simulink model "Model_Vehicle1D_Custom_24b"  (R2024b)
settings: Solver=VariableStepAuto  StartTime=0.0  StopTime=300  RelTol=1e-3
libraries: fl_lib x6, nesl_utility x4, sdl_lib x2
settings Model: Creator=isaacito  LastModifiedBy=isaacito
settings DataIOCC: DSMLogging=off
settings SimscapeCC: SimscapeLogType=all  SimscapeLogSimulationStatistics=on  SimscapeLogLimitData=off

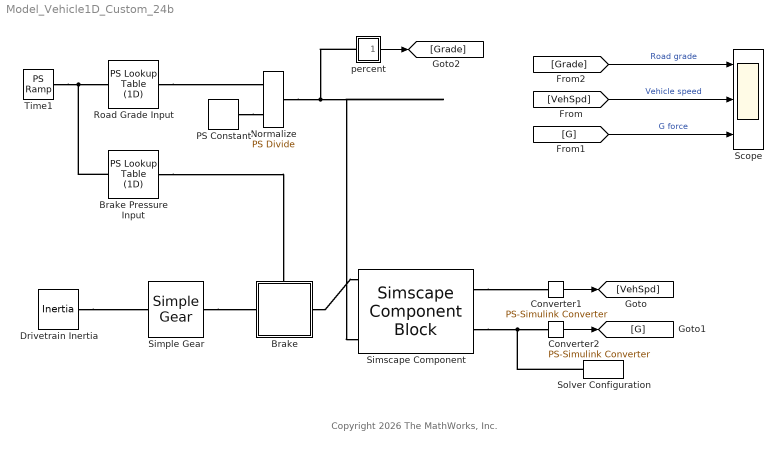
== system Model_Vehicle1D_Custom_24b ==
  note: Copyright 2026 The MathWorks, Inc.
  Brake : Subsystem
      settings: PortSchema="{\"entries\":[{\"content\":{\"sides\":[{\"content\":{\"connectorIds\":[\"LConn1\"]},\"type\":\"ConnectorPlacement.EquallySpacedRectSide\",\"uuid\":\"c6b073dd-2713-4a5b-85ee-4b5913294757\"},{\"content\":{\"connectorIds\":[\"RConn1\"],\"side\":\"RIGHT\"},\"type\":\"ConnectorPlacement.EquallySpacedRectSide\",\"uuid\":\"bfc45b1f-17ac-472b-87f9-2453469bccb5\"},{\"content\":{\"connectorIds\":[\"LConn2\"],\"side\":\"TOP\"},\"type\":\"ConnectorPlacement.EquallySpacedRectSide\",\"uuid\":\"4f05775c-3f1a-4bd9-8953-8138b3f9abd3\"}]},\"type\":\"ConnectorPlacement.EquallySpacedConnector\",\"uuid\":\"6aab441d-31a0-4c85-b942-993fc4aff852\"}],\"packageUris\":[\"http://schema.mathworks.com/mf0/Connector/R2020b\"],\"version\":\"1.0\"}"
  Brake Pressure Input : fl_lib/Physical Signals/Lookup Tables/PS Lookup Table (1D)  x=[0 1 2] s  f=[0 0 0] Pa  interp_method=simscape.enum.interpolation.smooth  extrap_method=simscape.enum.extrapolation.nearest
  Converter1 : nesl_utility/PS-Simulink Converter  PhysicalDomain=network_engine_domain  SubClassName=ps_output  LeftPortType=input  RightPortType=output  PseudoPeriodic=off  Frequencies=[]  VectorFormat=inherit  Unit=km/hr  AffineConversion=off
  Converter2 : nesl_utility/PS-Simulink Converter  PhysicalDomain=network_engine_domain  SubClassName=ps_output  LeftPortType=input  RightPortType=output  PseudoPeriodic=off  Frequencies=[]  VectorFormat=inherit  Unit=1  AffineConversion=off
  Drivetrain Inertia : fl_lib/Mechanical/Rotational Elements/Inertia  inertia=20*0.1^2 kg*m^2  num_ports=foundation.enum.numPorts2.one  w_specify=off  w_priority=High  w=0 rad/s  w_nominal_specify=off  w_nominal_value=1  w_nominal_unit=rad/s  t_specify=off  t_priority=None  t=0 N*m  t_nominal_specify=off  t_nominal_value=1  t_nominal_unit=N*m
  Normalize : fl_lib/Physical Signals/Functions/PS Divide
  PS Constant : fl_lib/Physical Signals/Sources/PS Constant  constant=100
      settings: AttributesFormatString=%<constant>
  Road Grade Input : fl_lib/Physical Signals/Lookup Tables/PS Lookup Table (1D)  Description=|  x=[0, 2.5, 5, 10, 25, 40, 80, 85, 90, 110, 130, 165, 200] s  f=[0, 0, 0, -10, -10, -10, 0, 0, 0, 5, 0, 0, 0]  interp_method=simscape.enum.interpolation.smooth  extrap_method=simscape.enum.extrapolation.nearest
      | % This text was automatically inserted by Signal Util.
      | % SignalDesignMatrixStart
      | [0 5 0; 10 40 -10; 80 90 0;
      |  110 nan 5; 130 200 0]
      | 
      | % SignalDesignMatrixEnd
  Scope : Scope  NumInputPorts=3
  Simple Gear : sdl_lib/Gears/Simple Gear  ratio=1/10  rotation_direction=sdl.enum.shaftOutputDirection.same  friction_model=sdl.enum.gear_efficiencies_load.off  T_noload=0.1 N*m  T_nom=5 N*m  efficiency_nom=0.8  efficiency=0.8  temperature_TLU=[280, 300, 320] K  load_TLU=[1, 5, 10] N*m  efficiency_TLU=[.95, .9, .85]  efficiency_TLU2=[.85, .8, .75; .95, .9, .85; .85, .8, .7]  w_thr=0.01 rad/s  pwr_thr=0.001 W  enable_backlash=false  hardstop_model=simscape.enum.hardstop.smooth  backlash_distance=1e-3 mm  r_base=0.1 m  transition=1e-4 mm  backlash_stiffness=1e6 N/m  backlash_damping=1e3 N*s/m  coeff_rest=0.7  v_tol=0.001 m/s  f_tol=0.001 N  mu_visc=[0, 0] N*m*s/rad  thermal_mass=50 J/K  temperature_specify=off  temperature_priority=High  temperature=300 K  temperature_nominal_specify=off  temperature_nominal_value=1  temperature_nominal_unit=K  x_backlash_specify=off  x_backlash_priority=None  x_backlash=0 mm  x_backlash_nominal_specify=off  x_backlash_nominal_value=1  x_backlash_nominal_unit=mm  f_hardstop_specify=off  f_hardstop_priority=None  f_hardstop=0 N  f_hardstop_nominal_specify=off  f_hardstop_nominal_value=1  f_hardstop_nominal_unit=N  v_backlash_specify=off  v_backlash_priority=None  v_backlash=0 m/s  v_backlash_nominal_specify=off  v_backlash_nominal_value=1  v_backlash_nominal_unit=m/s
      settings: AttributesFormatString=%<ratio>
  Simscape Component : SimscapeComponentBlock  SourceFile=Vehicle1D_Custom  ComponentPath=Vehicle1D_Custom  ComponentVariants="[\"Vehicle1D_Custom\"]"  ComponentVariantNames="[\"Vehicle1D_Custom\"]"  ClassName=Vehicle1D_Custom  SchemaVersion=1  grav=9.81 m/s^2  M_e=1500 kg  R_tire=0.3 m  A_rl=120 N  B_rl=0 N*hr/km  C_rl=0.03 N*hr^2/km^2  V_1=0.1 km/hr  w_1=0.1 rpm  V_x_specify=off  V_x_priority=High  V_x=0 km/hr  V_x_nominal_specify=off  V_x_nominal_value=1  V_x_nominal_unit=km/hr
      settings: CopyFcn=simscape.engine.sli.internal.componentblockcallback(gcbh,'COPY')  PreCopyFcn=simscape.engine.sli.internal.componentblockcallback(gcbh,'PRECOPY')  PreDeleteFcn=simscape.engine.sli.internal.componentblockcallback(gcbh,'PREDELETE')  InternalSimscapePortConfiguration="{\"Bottom\":[],\"Left\":[{\"id\":\"Axle\",\"label\":\"Axle\",\"type\":\"foundation.mechanical.rotational.rotational\"}],\"Right\":[{\"id\":\"v_out\",\"label\":\"V\",\"type\":\"output\"},{\"id\":\"G\",\"label\":\"G\",\"type\":\"output\"}],\"Top\":[{\"id\":\"brkF\",\"label\":\"Brake\",\"type\":\"input\"},{\"id\":\"grade_norm\",\"label\":\"Grade\",\"type\":\"input\"}]}"
      mask Type: Custom Longitudinal Vehicle
  Solver Configuration : nesl_utility/Solver Configuration  PhysicalDomain=network_engine_domain  SubClassName=solver  LeftPortType=input  RightPortType=generic  Tones=[]  Harmonics=[]  SimulateNoise=off  Profile=off  UseLocalSampling=off  EnableSwitchedLinearOptims=on  FrequencyDomain=off  UseCCode=off  RelTol=0.001  AbsTol=0.001  MinStep=1e-09  ToWorkspace=off  RevertToSquareIcSolve=off  NumHomotopyIterations=100  PhasorMode=off  PhasorModeNumHarmonics=1  ConsistencySolver=NEWTON_XTOL_AFTER_FTOL  IndexReductionMethod=DerivativeReplacement  DoDC=off  ResidualTolerance=1e-09  ConsistencyTolSource=GLOBAL  ConsistencyAbsTol=0.001  ConsistencyRelTol=0.001  ConsistencyTolFactor=0.001  UseLocalSolver=off  LocalSolverChoice=NE_BACKWARD_EULER_ADVANCER  ResolveIndetEquations=on  FunctionEvalNumThread=1  LocalSolverSampleTime=0.001  DoFixedCost=off  MaxNonlinIter=3  MaxModeIter=2  ComputeImpulses=off  ImpulseIterations=2  LinearAlgebra=auto  LinearAlgebraNumThread=0  EquationFormulation=NE_TIME_EF  DelaysMemoryBudget=1024  AutomaticFiltering=on  FilteringTimeConstant=0.001  PartitionStorageMethod=AS_NEEDED  PartitionMemoryBudget=1024  PartitionMethod=ROBUST  MultibodyUseLocalSolver=off  MultibodyLocalSolverChoice=ODE1  MultibodyLocalSolverSampleTime=0.001
      settings: AttributesFormatString=Local solver: %<UseLocalSolver>
  Time1 : fl_lib/Physical Signals/Sources/PS Ramp  slope=1  start_time=0 s  initial_output=0 s
  percent : Subsystem
  wires:
  [VehSpd] -> Scope/2  "Vehicle speed"
  Converter1/1 -> [VehSpd]
  Converter2/1 -> [G]
  [G] -> Scope/3  "G force"
  [Grade] -> Scope/1  "Road grade"
  percent/1(Out1) -> [Grade]
  connections:
  Simscape Component/RConn2 -- Solver Configuration/RConn1 -- Converter2/LConn1
  Brake/RConn1 -- Simscape Component/LConn1
  Simple Gear/RConn1 -- Brake/LConn1
  Brake Pressure Input/RConn1 -- Brake/LConn2
  Time1/RConn1 -- Brake Pressure Input/LConn1 -- Road Grade Input/LConn1
  Drivetrain Inertia/LConn1 -- Simple Gear/LConn1
  Simscape Component/RConn1 -- Converter1/LConn1
  Road Grade Input/RConn1 -- Normalize/LConn1
  PS Constant/RConn1 -- Normalize/LConn2
  Normalize/RConn1 -- percent/LConn1 -- Simscape Component/LConn3

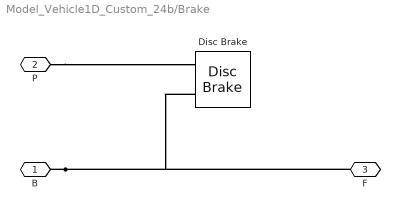
== system Model_Vehicle1D_Custom_24b/Brake ==
  Disc Brake : sdl_lib/Brakes & Detents/Rotational/Disc Brake  r_mean=150 mm  bore=10 mm  n_pads=2  thermal_port=simscape.enum.thermaleffects.omit  mu_static=0.9  mu_coulomb=0.7  temperature_TLU=[280, 300, 320] K  mu_static_TLU=[.9, .8, .7]  mu_coulomb_TLU=[.8, .7, .6]  brkwy_vel=0.1 rad/s  visc_coef=0 N*m*s/rad  thermal_mass=50 kJ/K  temperature_specify=off  temperature_priority=High  temperature=300 K  temperature_nominal_specify=off  temperature_nominal_value=1  temperature_nominal_unit=K
  B : PMIOPort  Side=Left
  P : PMIOPort  Port=2  Side=Left
  F : PMIOPort  Port=3  Side=Right
  connections:
  B/RConn1 -- Disc Brake/LConn2 -- F/RConn1
  P/RConn1 -- Disc Brake/LConn1

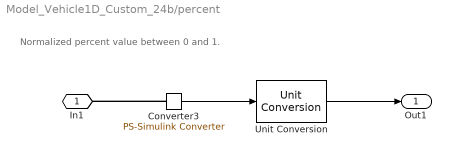
== system Model_Vehicle1D_Custom_24b/percent ==
  note: Normalized percent value between 0 and 1.
  Converter3 : nesl_utility/PS-Simulink Converter  PhysicalDomain=network_engine_domain  SubClassName=ps_output  LeftPortType=input  RightPortType=output  PseudoPeriodic=off  Frequencies=[]  VectorFormat=inherit  Unit=1  AffineConversion=off
  Unit Conversion : UnitConversion
  In1 : PMIOPort  Side=Left
  Out1 : Outport  Unit=%
  wires:
  Unit Conversion/1 -> Out1/1
  Converter3/1 -> Unit Conversion/1
  connections:
  Converter3/LConn1 -- In1/RConn1
